simulink model "Foc_model_Matlab_obs"  (R2024b)
settings: Solver=FixedStepDiscrete  StartTime=0.0  StopTime=5  RelTol=1e-3  EnableMultiTasking=on
PreLoadFcn:
  | mcb_pmsm_foc_hall_S32K144EVB_data;
InitFcn:
  | mbd_s32k_consistency_checks(bdroot(gcs));
model workspace (MAT data in the model file):
  IDC_OVERCURRENT = Simulink.Parameter
  IDC_OVERCURRENT.Value = 2.3
  IDC_OVERCURRENT.Complexity = 'real'
  IDC_OVERCURRENT.Dimensions = [1 1]
  IDC_OVERCURRENT.DataType = 'single'
  VDC_OVERVOLTAGE = Simulink.Parameter
  VDC_OVERVOLTAGE.Value = 16
  VDC_OVERVOLTAGE.Complexity = 'real'
  VDC_OVERVOLTAGE.Dimensions = [1 1]
  VDC_OVERVOLTAGE.DataType = 'single'
  VDC_UNDERVOLTAGE = Simulink.Parameter
  VDC_UNDERVOLTAGE.Value = 8
  VDC_UNDERVOLTAGE.Complexity = 'real'
  VDC_UNDERVOLTAGE.Dimensions = [1 1]
  VDC_UNDERVOLTAGE.DataType = 'single'
undefined symbols (not defined in the file): DiscIntNeverNeededParam, External, inverter, Kcd, Kcq, Kid, Kiq, Kis, LQFP, mcb_isCodeGenVar, mcb_isSimVar, One, PI_params, pmsm, PU_System, Shot, sigbuilder_block, TRGMUX_PDB_TRIG, Ts, Ts_motor, Ts_simulink, Ts_speed
libraries: mbd_s32k1xx_ec_toolbox x35, mcbcontrolslib x8, simulink x6, mbd_msd_ec_toolbox x5, mcbpositiondecoderlib x3, hdlsllib x2, slpidlib x1, mcbsensorlessestimatorlib x1, mcbplantlib x1, autolibpmsmexterior x1, SignalEditorBlockLib x1
(part 1 of 2)
Description:
  | Field-Oriented Control for PMSM with Hall sensor with MTRDEVSPNK144.
  | This Simulink model is designed to work with Linix 45ZWN24-40 Motor and validate
  | that the motor can be rotated in closed loop with Hall sensor in Mathworks model from Motor Control Blockset.
  | The main scope of the model is to validate that the motor can run using Field-Oriented Control with Hall sensor.
  | 
  | FEATURES:
  | - Use FreeMASTER pannel to control the speed,
  | - Measure the 3-phase sinusoidal currents with PWM-PDB-ADC synchronization,
  | - Measure the DC bus voltage and current with PWM-PDB-ADC synchronization,
  | - PI Speed, Flux and Torque Controllers, position observer using Hall sensor.
  | 
  | HW SETUP:
  | - Configure S32K144 board supply voltage: J107:2-3(over USB),
  | - Configure J9,J10 and J11 on MotorGD: 2-3 (mode PMSM),
  | - Rotate trimmer resistor R72 (placed Devkit-MotorGD) counter-clockwise at maximum,
  | - Connect the motor phases to MotorGD J13 connector
  |   (i.e. Linix 45ZWN24-40: phA-white/phB-blue/phC-green),
  | - Power on the kit via J7 connector with 12Vdc.
  | 
  | VALIDATION:
  | - Run "mcb_pmsm_hall_offset_S32K144EVB_NXP.mdl" model to find out the position offset and
  | update it in "mcb_pmsm_foc_hall_S32K144EVB_data.m" script, run this script,
  | - Build/Simulate the model,
  | - After reset or power on, the Green LED shall be ON,
  | - In case of a FAULT the Red LED will be ON,
  | - Open FreeMASTER project and connect to the target.
  | - The initial speed command is set to 450rpm and can be changed from FreeMaster project.
  | - Click on the ON/OFF button to start then the speed of the motor it can be
  | changed using Speed gauge.
  | 
  | NOTE:
  | - In case of fault (RED LED is ON), the remove fault cause and press RESET button
  | 
  | Copyright (c) 2021 NXP
  | version 1.0.0
settings Model: Creator=nxf40284  LastModifiedBy=diego
settings SolverCC: AlgebraicLoopSolver=TrustRegion
settings DataIOCC: ExternalInput=off  InitialState=off  LimitDataPoints=on  SaveFormat=Array  SaveOutput=off  SaveTime=off  ReturnWorkspaceOutputs=off
settings OptimizationCC: DefaultParameterBehavior=Inlined  UseFloatMulNetSlope=on  DefaultUnderspecifiedDataType=single  UseSpecifiedMinMax=on  EnhancedBackFolding=on  PassReuseOutputArgsAs=Individual arguments  ZeroExternalMemoryAtStartup=off  ZeroInternalMemoryAtStartup=off  NoFixptDivByZeroProtection=on  EfficientFloat2IntCast=on  EfficientTunableParamExpr=on
settings DebuggingCC: AlgebraicLoopMsg=error  ArtificialAlgebraicLoopMsg=error  SolverPrmCheckMsg=warning  InheritedTsInSrcMsg=none  MultiTaskDSMMsg=none  MultiTaskCondExecSysMsg=none  TasksWithSamePriorityMsg=none  SigSpecEnsureSampleTimeMsg=none  ParameterPrecisionLossMsg=none  ParameterTunabilityLossMsg=error  FcnCallInpInsideContextMsg=warning  UnconnectedInputMsg=error  UnconnectedOutputMsg=error  UnconnectedLineMsg=error  AllowSymbolicDim=off  StateNameClashWarn=warning  SFUnexpectedBacktrackingDiag=warning  SFNoUnconditionalDefaultTransitionDiag=warning  SFExecutionAtInitializationDiag=none  ArithmeticOperatorsInVariantConditions=warning
settings HardwareCC: ProdBitPerPointer=32  ProdBitPerSizeT=32  ProdBitPerPtrDiffT=32  ProdLargestAtomicInteger=Long  ProdLargestAtomicFloat=Double  ProdWordSize=32  ProdHWDeviceType=ARM Compatible->ARM Cortex
settings ModelReferenceCC: EnableRefExpFcnMdlSchedulingChecks=on
settings SFSimCC: MATLABDynamicMemAlloc=off
settings RTWCC: Description=Model Based Design Toolbox S32K1xx Code Generation Target  SystemTargetFile=mbd_s32k.tlc  MakeCommand=mbd_s32k_make_rtw COPY_MDLREF_INCLUDES=0  TemplateMakefile=mbd_s32k.tmf  GenerateReport=on  IncludeHyperlinkInReport=on  GenerateTraceInfo=on  GenerateTraceReport=on  GenerateTraceReportSl=on  GenerateTraceReportSf=on  GenerateTraceReportEml=on  GPUComputeCapability=3.5
settings CodeAppCC: ForceParamTrailComments=on  IgnoreCustomStorageClasses=off  OperatorAnnotations=on  SimulinkDataObjDesc=on  SFDataObjDesc=on  InsertBlockDesc=on  StateflowObjectComments=on
settings STFCustomTargetCC: MultiwordLength=256  CombineOutputUpdateFcns=on  ERTCustomFileBanners=on  SupportContinuousTime=off  SupportNonInlinedSFcns=off  RemoveResetFunc=on  MATLABClassNameForMDSCustomization=Simulink.SoftwareTarget.ERTCustomization  SystemTargetFile=mbd_s32k.tlc
settings ERTTargetCC: ParMdlRefBuildCompliant=off  CompOptLevelCompliant=off  ConcurrentExecutionCompliant=off  ModelStepFunctionPrototypeControlCompliant=off  CPPClassGenCompliant=off  UseToolchainInfoCompliant=off  ERTSrcFileBannerTemplate=mbd_ert_code_template.cgt  ERTHdrFileBannerTemplate=mbd_ert_code_template.cgt  ERTDataSrcFileTemplate=mbd_ert_code_template.cgt  ERTDataHdrFileTemplate=mbd_ert_code_template.cgt  ERTCustomFileTemplate=example_file_process.tlc  ConvertIfToSwitch=off  SuppressUnreachableDefaultCases=off  DynamicArrayContainerType=coder::array

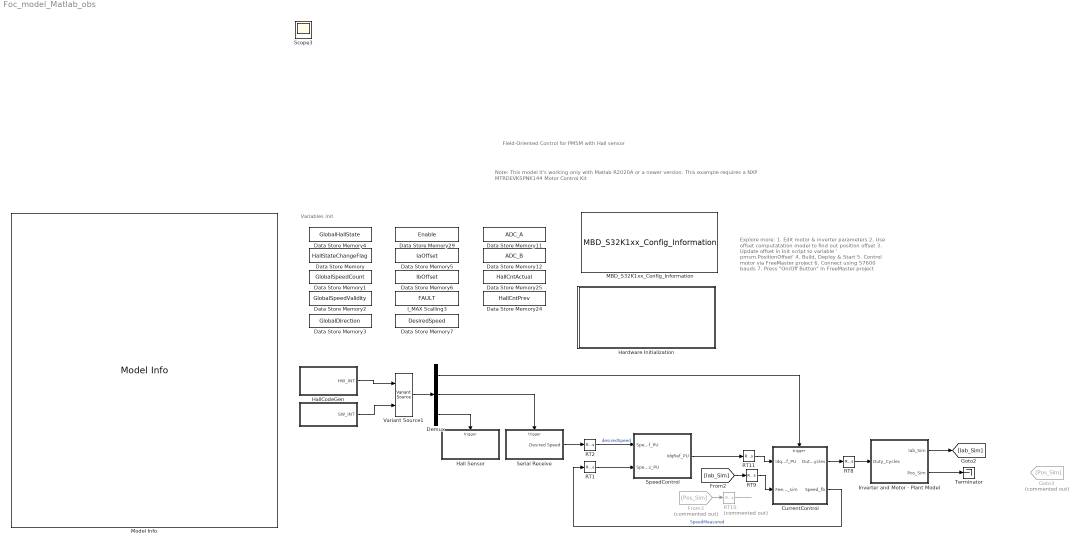
== system Foc_model_Matlab_obs ==
  note: Variables init
  note: Field-Oriented Control for PMSM with Hall sensor
  note: Explore more:
      | 1. Edit motor & inverter parameters
      | 2. Use offset computatation model to
      | find out position offset
      | 3. Update offset in Init script to variable ' pmsm.PositionOffset'
      | 4. Build, Deploy & Start
      | 5. Control motor via FreeMaster project
      | 6. Connect using 57600 bauds
      | 7. Press "On/Off Button" in FreeMaster project
  note: Note: This model it's working only with Matlab R2020A or a newer version.
      | This example requires a NXP MTRDEVKSPNK144 Motor Control Kit
  " " : Subsystem
  CurrentControl : Subsystem
      settings: RTWSystemCode=Nonreusable function  RTWFcnNameOpts=Use subsystem name
  Data Store Memory : DataStoreMemory  DataStoreName=HallStateChangeFlag  ShowAdditionalParam=off  OutDataTypeStr=uint16
  Data Store Memory1 : DataStoreMemory  DataStoreName=GlobalSpeedCount  ShowAdditionalParam=off  OutDataTypeStr=uint16
  Data Store Memory11 : DataStoreMemory  DataStoreName=ADC_A  ShowAdditionalParam=off
  Data Store Memory12 : DataStoreMemory  DataStoreName=ADC_B  ShowAdditionalParam=off
  Data Store Memory2 : DataStoreMemory  DataStoreName=GlobalSpeedValidity  ShowAdditionalParam=off  OutDataTypeStr=uint16
  Data Store Memory24 : DataStoreMemory  DataStoreName=HallCntPrev  ReadBeforeWriteMsg=warning  WriteAfterWriteMsg=warning  WriteAfterReadMsg=warning  ShowAdditionalParam=off  OutDataTypeStr=uint16
  Data Store Memory25 : DataStoreMemory  DataStoreName=HallCntActual  ReadBeforeWriteMsg=warning  WriteAfterWriteMsg=warning  WriteAfterReadMsg=warning  ShowAdditionalParam=off  OutDataTypeStr=uint16
  Data Store Memory29 : DataStoreMemory  DataStoreName=Enable  ShowAdditionalParam=off  OutDataTypeStr=boolean
  Data Store Memory3 : DataStoreMemory  DataStoreName=GlobalDirection  ShowAdditionalParam=off  OutDataTypeStr=int16
  Data Store Memory4 : DataStoreMemory  DataStoreName=GlobalHallState  ShowAdditionalParam=off  OutDataTypeStr=uint32
  Data Store Memory5 : DataStoreMemory  DataStoreName=IaOffset  InitialValue=inverter.CtSensAOffset  ShowAdditionalParam=off  OutDataTypeStr=single
  Data Store Memory6 : DataStoreMemory  DataStoreName=IbOffset  InitialValue=inverter.CtSensBOffset  ShowAdditionalParam=off  OutDataTypeStr=single
  Data Store Memory7 : DataStoreMemory  DataStoreName=DesiredSpeed  ReadBeforeWriteMsg=warning  WriteAfterWriteMsg=warning  WriteAfterReadMsg=warning  InitialValue=450  ShowAdditionalParam=off  OutDataTypeStr=single
  Demux : Demux  Outputs=3
  From3 : From  Commented=on  GotoTag=Pos_Sim
  Goto3 : Goto  Commented=on  GotoTag=Pos_Sim
  Hall Sensor : Subsystem
  HallCodeGen : Subsystem
  Hardware Initialization : Subsystem  Priority=2
  I_MAX Scalling3 : DataStoreMemory  Priority=0  DataStoreName=FAULT  ReadBeforeWriteMsg=warning  WriteAfterWriteMsg=warning  WriteAfterReadMsg=warning  ShowAdditionalParam=off  OutDataTypeStr=boolean
  Inverter and Motor - Plant Model : Subsystem
  MBD_S32K1xx_Config_Information : mbd_s32k1xx_ec_toolbox/MBD_S32K1xx_Config_Information  Priority=1  mbdt_ver=0  disp_str=|  config_params=[]  mcu_target_name=S32K144  mcu_target_package=100-LQFP  mcu_target_sram_size=64KB  mcu_system_clock_freq=80  mcu_xtal_freq=External 8  mcu_steptick_timer=LPIT Channel 0  mcu_steptick_prio=15  ds_import_enable=on  target_compiler=GCC  target_memory=FLASH  gcc_target_compile_opts=-mcpu=cortex-m4 -mthumb -mfloat-abi=hard -mfpu=fpv4-sp-d16 -O1 -g -gstrict-dwarf  gcc_target_assemble_opts=-mcpu=cortex-m4 -mthumb -mfloat-abi=hard -mfpu=fpv4-sp-d16 -g  gcc_target_link_opts=-mcpu=cortex-m4 -mthumb -mfloat-abi=hard -mfpu=fpv4-sp-d16  gcc_target_default_lcf=on  gcc_target_user_lcf=S32K144_64_flash.ld  ghs_target_compile_opts=-cpu=cortexm4f -thumb -DARM_MATH_CM4 -fpu=vfpv4_d16 -fsingle -Ogeneral -Wundef -Wimplicit-int -Wshadow -Wtrigraphs --no_commons --gnu_asm -gnu99 -gdwarf-2 -G  ghs_target_assemble_opts=-cpu=cortexm4f -fpu=vfpv4_d16  ghs_target_link_opts=-cpu=cortexm4f -thumb -fpu=vfpv4_d16  ghs_target_default_lcf=on  ghs_target_user_lcf=S32K144_64_flash.ld  iar_target_compile_opts=--cpu=Cortex-M4F --thumb --fpu=VFPv4_sp -Ol -e --debug --dlib_config normal  iar_target_assemble_opts=--cpu Cortex-M4F --thumb --fpu VFPv4_sp  iar_target_link_opts=--no_exceptions --vfe --inline  iar_target_default_lcf=on  iar_target_user_lcf=S32K144_64_flash.icf  pil_download_enable=off  rbl_download_enable=on  rbl_start_delay=5000  rbl_download_interface=OpenSDA  rbl_restart_request=off  rbl_com_port=Custom  rbl_com_port_custom=COM1  pil_download_rate=57600  pil_opensda_drive=Custom  pil_opensda_drive_custom=D  pil_uart_instance=1  pil_uart_rx=PTC6: [LPUART1_RX | Receive]  pil_uart_tx=PTC7: [LPUART1_TX | Transmit]  FTM_PWM_PcrCheckEnDis=on  FTM_Input_Edge_Inputs_PcrCheckEnDis=on  FTM_Dual_Edge_Inputs_PcrCheckEnDis=on  FTM_Quadrature_Inputs_PcrCheckEnDis=on  FTM_Hall_Sensor_Inputs_PcrCheckEnDis=on  LPTMR_PcrCheckEnDis=on  PIT_PcrCheckEnDis=on  RTC_PcrCheckEnDis=on  FlexCAN_PcrCheckEnDis=on  LIN_PcrCheckEnDis=on  FlexIO_PcrCheckEnDis=on  LPI2C_PcrCheckEnDis=on  LPSPI_PcrCheckEnDis=on  LPUART_PcrCheckEnDis=on  CMP_PcrCheckEnDis=on  GPIO_OutputPcrCheckEnDis=on  GPIO_InputPcrCheckEnDis=on  SBC_PcrCheckEnDis=on  BMS_PcrCheckEnDis=on  AMMCLIB_PcrCheckEnDis=on  FM_PcrCheckEnDis=on  Profile_PcrCheckEnDis=on  ConfigParams_PcrCheckEnDis=on  ModelRef_PcrCheckEnDis=on  PDB0_PcrCheckEnDis=on  CSEc_PcrCheckEnDis=on  eDMA_PcrCheckEnDis=on  FLASH_PcrCheckEnDis=on  ADC_PcrCheckEnDis=on  WDOG_PcrCheckEnDis=on
      | Target : S32K144-64KB_SRAM
      | Package : 100-pin
      | System clock : 80 MHz
      | XTAL clock : External 8 MHz
      | Compiler : IAR
      | Target Type : FLASH
      | Download Code after build : off
      | Step Tick Interrupt Priority : 15
  Model Info : simulink/Model-Wide Utilities/Model Info  Frame=off  DisplayStringWithTags=|  HorizontalTextAlignment=Left  LeftAlignmentValue=0.02
      | Model Name: %<ModelName>
      | 
      | Description: %<Description>
  RT1 : RateTransition  Priority=2  Deterministic=off  OutPortSampleTime=Ts_speed
  RT10 : RateTransition  Commented=on  Deterministic=off  OutPortSampleTime=Ts
  RT11 : RateTransition  Deterministic=off  OutPortSampleTime=Ts
  RT2 : RateTransition  Priority=1  Deterministic=off  OutPortSampleTime=Ts_speed
  RT8 : RateTransition  Deterministic=off
  RT9 : RateTransition  Deterministic=off  OutPortSampleTime=Ts
  Serial Receive : Subsystem  SystemSampleTime=1e-3
  SpeedControl : Subsystem  TreatAsAtomicUnit=on  SystemSampleTime=Ts_speed
      settings: RTWSystemCode=Nonreusable function  RTWFcnNameOpts=Use subsystem name
  Terminator : Terminator
  Variant Source1 : VariantSource
  Scope3 : Scope
  wires:
  " "/1(SW_INT) -> Variant Source1/2
  HallCodeGen/1(HW_INT) -> Variant Source1/1
  [Iab_Sim] -> RT9/1
  Serial Receive/1(Desired Speed) -> RT2/1
  RT9/1 -> CurrentControl/2(Feedbacks_sim)
  RT11/1 -> CurrentControl/1(Idq_ref_PU)
  From3/1 -> RT10/1
  RT10/1 -> ?
  SpeedControl/1(IdqRef_PU) -> RT11/1
  RT2/1 -> SpeedControl/1(Speed_Ref_PU)  "desiredSpeed"
  CurrentControl/1(Duty Cycles) -> RT8/1
  RT8/1 -> Inverter and Motor - Plant Model/1(Duty_Cycles)
  Inverter and Motor - Plant Model/2(Pos_Sim) -> Terminator/1
  Inverter and Motor - Plant Model/1(Iab_Sim) -> [Iab_Sim]
  RT1/1 -> SpeedControl/2(Speed_Meas_PU)
  CurrentControl/2(Speed_fb) -> RT1/1  "SpeedMeasured"
  Variant Source1/1 -> Demux/1
  Demux/3 -> Hall Sensor/Trigger
  Demux/2 -> Serial Receive/Trigger
  Demux/1 -> CurrentControl/Trigger

== system Foc_model_Matlab_obs/  ==
  CurrentController_INT : simulink/Ports & Subsystems/Function-Call Generator  sample_time=Ts  numberOfIterations=1  DisallowWideOutput=off
  Hall_INT : simulink/Ports & Subsystems/Function-Call Generator  sample_time=Ts  numberOfIterations=1  DisallowWideOutput=off
  Mux : Mux  Inputs=3
  SCI_Rx_INT : simulink/Ports & Subsystems/Function-Call Generator  sample_time=Ts  numberOfIterations=1  DisallowWideOutput=off
  SW_INT : Outport
  wires:
  Mux/1 -> SW_INT/1
  CurrentController_INT/1 -> Mux/1
  Hall_INT/1 -> Mux/3
  SCI_Rx_INT/1 -> Mux/2

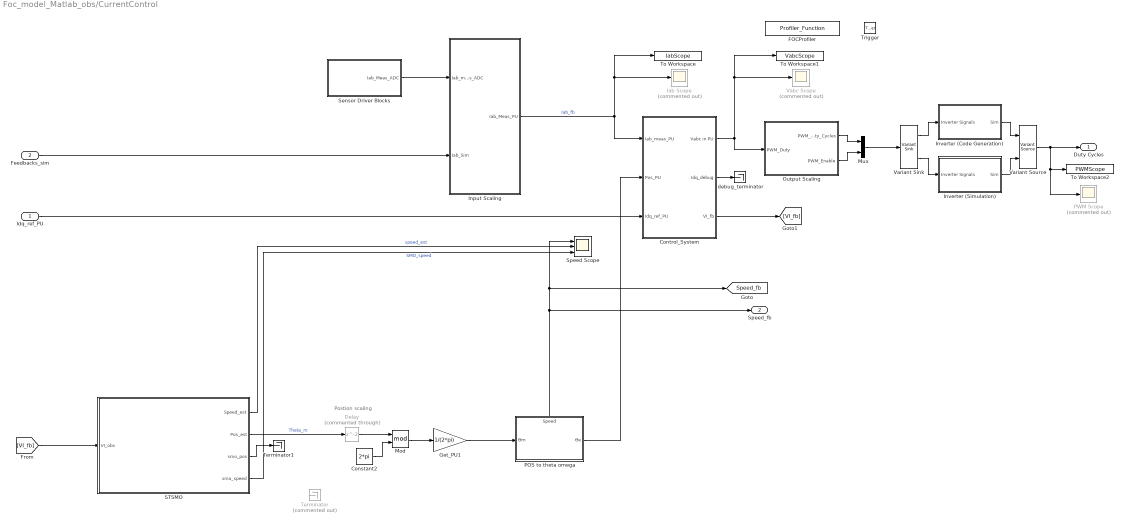
== system Foc_model_Matlab_obs/CurrentControl ==
  note: Postion scaling
  Idq_ref_PU : Inport
  Feedbacks_sim : Inport  Port=2
  Trigger : TriggerPort  TriggerType=function-call  VariantControl=Variant
  Constant2 : Constant  Value=2*pi  OutDataTypeStr=single  SampleTime=-1
  Control_System : Subsystem  Priority=3
  Delay : Delay  Commented=through
  FOCProfiler : mbd_s32k1xx_ec_toolbox/Utility Blocks/Profiler_Function  profile_indx=0
  Get_PU1 : Gain  Gain=1/(2*pi)  OutDataTypeStr=dataType  RndMeth=Simplest
  Iab Scope : Scope  Commented=on
  Input Scaling : Subsystem
  Inverter (Code Generation) : Subsystem  Priority=5
  Inverter (Simulation) : Subsystem
  Mod : Math  Operator=mod
  Mux : Mux  Inputs=2
  Output Scaling : Subsystem  Priority=4
  POS to theta omega : Subsystem
      settings: PortSchema="{\"entries\":[{\"content\":{\"sides\":[{\"content\":{\"connectorIds\":[\"In1\"]},\"type\":\"ConnectorPlacement.EquallySpacedRectSide\",\"uuid\":\"835816d9-4aa8-456c-963d-288b2d91bd0d\"},{\"content\":{\"connectorIds\":[\"Out1\"],\"side\":\"RIGHT\"},\"type\":\"ConnectorPlacement.EquallySpacedRectSide\",\"uuid\":\"100271e0-f614-4ef1-83bc-12c7604e80ba\"},{\"content\":{\"connectorIds\":[\"Out2\"],\"side\":\"TOP\"},\"type\":\"ConnectorPlacement.EquallySpacedRectSide\",\"uuid\":\"e3f4bec2-de67-41f7-95c5-b7e3793c521c\"}]},\"type\":\"ConnectorPlacement.EquallySpacedConnector\",\"uuid\":\"b67e7fce-f36c-4173-939b-340321a87f64\"}],\"packageUris\":[\"http://schema.mathworks.com/mf0/Connector/R2020b\"],\"version\":\"1.0\"}"
  PWM Scope : Scope  Commented=on
  STSMO : Subsystem
  Sensor Driver Blocks : Subsystem  Variant=on
  Speed Scope : Scope  NumInputPorts=3
  Terminator : Terminator  Commented=on
  Terminator1 : Terminator
  To Workspace : ToWorkspace  VariableName=IabScope  SaveFormat=Structure With Time  SampleTime=-1
  To Workspace1 : ToWorkspace  VariableName=VabcScope  SaveFormat=Structure With Time  SampleTime=-1
  To Workspace2 : ToWorkspace  VariableName=PWMScope  SaveFormat=Structure With Time  SampleTime=-1
  Vabc Scope : Scope  Commented=on
  Variant Sink : VariantSink
  Variant Source : VariantSource
  debug_terminator : Terminator
  Duty Cycles : Outport  InitialOutput=0  VectorParamsAs1DForOutWhenUnconnected=off
  Speed_fb : Outport  Port=2  InitialOutput=0  VectorParamsAs1DForOutWhenUnconnected=off
  tag scope: Speed_fb=global
  wires:
  Sensor Driver Blocks/1(Iab_Meas_ADC) -> Input Scaling/1(Iab_meas_ADC)
  Control_System/1(Vabc in PU) -> Output Scaling/1(PWM_Duty), To Workspace1/1, Vabc Scope/1
  Idq_ref_PU/1 -> Control_System/3(Idq_ref_PU)
  Input Scaling/1(Iab_Meas_PU) -> To Workspace/1, Iab Scope/1, Control_System/1(Iab_meas_PU)  "Iab_fb"
  Feedbacks_sim/1 -> Input Scaling/2(Iab_Sim)
  Output Scaling/1(PWM_Duty_Cycles) -> Mux/1
  Output Scaling/2(PWM_Enable) -> Mux/2
  Control_System/2(Idq_debug) -> debug_terminator/1
  Variant Sink/1 -> Inverter (Code Generation)/1(Inverter Signals)
  Inverter (Code Generation)/1(Sim) -> Variant Source/1
  Inverter (Simulation)/1(Sim) -> Variant Source/2
  Variant Sink/2 -> Inverter (Simulation)/1(Inverter Signals)
  Mux/1 -> Variant Sink/1
  Variant Source/1 -> To Workspace2/1, PWM Scope/1, Duty Cycles/1
  Control_System/3(VI_fb) -> [VI_fb]
  [VI_fb] -> STSMO/1(VI_obs)
  STSMO/3(smo_pos) -> Terminator1/1
  STSMO/4(smo_speed) -> Speed Scope/3  "SMO_speed"
  STSMO/1(Speed_est) -> Speed Scope/2  "speed_est"
  Constant2/1 -> Mod/2
  STSMO/2(Pos_est) -> Delay/1  "Theta_m"
  Mod/1 -> Get_PU1/1
  Get_PU1/1 -> POS to theta omega/1(ϴm)
  POS to theta omega/1(ϴe) -> Control_System/2(Pos_PU)
  POS to theta omega/2(Speed) -> Speed Scope/1, [Speed_fb], Speed_fb/1
  Delay/1 -> Mod/1

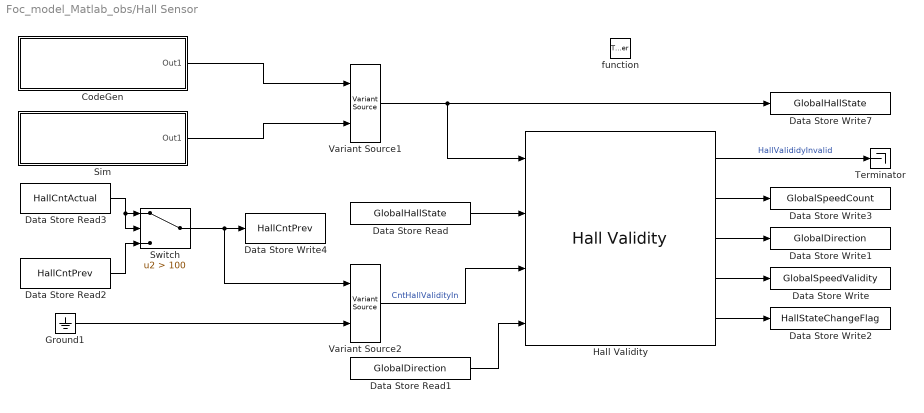
== system Foc_model_Matlab_obs/Hall Sensor ==
  function : TriggerPort  TriggerType=function-call  VariantControl=Variant
  CodeGen : Subsystem
  Data Store Read : DataStoreRead  Priority=1  DataStoreName=GlobalHallState  IndexOptions=Index vector (dialog)  Indices=1  OutputSizes=1
  Data Store Read1 : DataStoreRead  DataStoreName=GlobalDirection  IndexOptions=Index vector (dialog)  Indices=1  OutputSizes=1
  Data Store Read2 : DataStoreRead  DataStoreName=HallCntPrev  IndexOptions=Index vector (dialog)  Indices=1  OutputSizes=1
  Data Store Read3 : DataStoreRead  DataStoreName=HallCntActual  IndexOptions=Index vector (dialog)  Indices=1  OutputSizes=1
  Data Store Write : DataStoreWrite  DataStoreName=GlobalSpeedValidity  IndexOptions=Index vector (dialog)  Indices=1  OutputSizes=1
  Data Store Write1 : DataStoreWrite  DataStoreName=GlobalDirection  IndexOptions=Index vector (dialog)  Indices=1  OutputSizes=1
  Data Store Write2 : DataStoreWrite  DataStoreName=HallStateChangeFlag  IndexOptions=Index vector (dialog)  Indices=1  OutputSizes=1
  Data Store Write3 : DataStoreWrite  DataStoreName=GlobalSpeedCount  IndexOptions=Index vector (dialog)  Indices=1  OutputSizes=1
  Data Store Write4 : DataStoreWrite  DataStoreName=HallCntPrev  IndexOptions=Index vector (dialog)  Indices=1  OutputSizes=1
  Data Store Write7 : DataStoreWrite  Priority=2  DataStoreName=GlobalHallState  IndexOptions=Index vector (dialog)  Indices=1  OutputSizes=1
  Ground1 : Ground
  Hall Validity : mcbpositiondecoderlib/Hall Validity  hallSequence=CBA  sequence=[6,4,5,1,3,2]  CounterSize=16 bits
  Sim : Subsystem
  Switch : Switch  Criteria=u2 > Threshold  Threshold=100  SaturateOnIntegerOverflow=off  InputSameDT=off
  Terminator : Terminator
  Variant Source1 : VariantSource
  Variant Source2 : VariantSource
  wires:
  Hall Validity/3 -> Data Store Write1/1
  Hall Validity/5 -> Data Store Write2/1
  Hall Validity/4 -> Data Store Write/1
  Data Store Read1/1 -> Hall Validity/4
  Hall Validity/2 -> Data Store Write3/1
  Data Store Read/1 -> Hall Validity/2
  Hall Validity/1 -> Terminator/1  "HallValididyInvalid"
  Variant Source1/1 -> Hall Validity/1, Data Store Write7/1
  Ground1/1 -> Variant Source2/2
  Switch/1 -> Variant Source2/1, Data Store Write4/1
  Sim/1(Out1) -> Variant Source1/2
  CodeGen/1(Out1) -> Variant Source1/1
  Data Store Read2/1 -> Switch/3
  Data Store Read3/1 -> Switch/2, Switch/1
  Variant Source2/1 -> Hall Validity/3  "CntHallValidityIn"

== system Foc_model_Matlab_obs/HallCodeGen ==
  Data Store Write1 : DataStoreWrite  Priority=1  DataStoreName=HallCntActual  IndexOptions=Index vector (dialog)  Indices=1  OutputSizes=1
  FTM_Hall_Sensor : mbd_s32k1xx_ec_toolbox/Motor Control Blocks/FTM Blocks/FTM_Hall_Sensor  Priority=1  e_mode=Rising or Falling  prescaler=128  max_period=0.10486  isrlevel=5  mcuTargetUpdate=on  filter_en=off  filter_value=0  pinFtm1Ch1=PTA1: [FTM1_CH1 | FTM Channel]  pinFtm2Ch0=PTD10: [FTM2_CH0 | FTM Channel]  pinFtm2Ch1=PTD11: [FTM2_CH1 | FTM Channel]
  Mux : Mux  Inputs=3
  SCI_Rx_INT : simulink/Ports & Subsystems/Function-Call Generator  sample_time=0.1  numberOfIterations=1  DisallowWideOutput=off
  Subsystem2 : Subsystem  TreatAsAtomicUnit=on
  HW_INT : Outport
  wires:
  FTM_Hall_Sensor/2 -> Data Store Write1/1  "CntHall"
  Mux/1 -> HW_INT/1
  FTM_Hall_Sensor/1 -> Mux/3
  Subsystem2/1(FcnCall) -> Mux/1
  SCI_Rx_INT/1 -> Mux/2

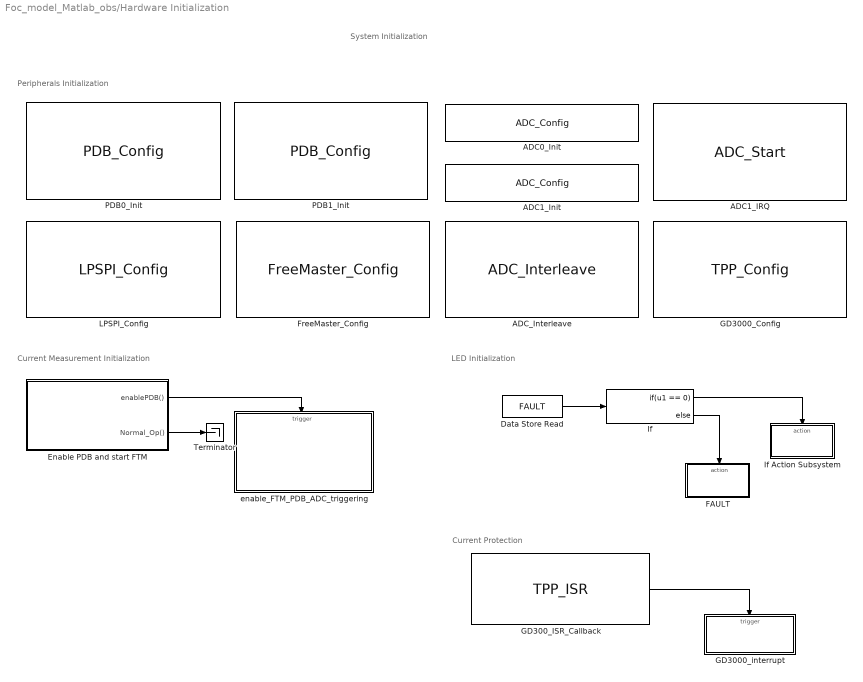
== system Foc_model_Matlab_obs/Hardware Initialization ==
  note: Peripherals Initialization
  note: System Initialization
  note: Current Measurement Initialization
  note: LED Initialization
  note: Current Protection
  ADC0_Init : mbd_s32k1xx_ec_toolbox/Motor Control Blocks/ADC Blocks/ADC_Config  Priority=3  instance=0  mode=12-bit conversion  smplts=2  adiclk=alternate clock 1  adiv=input clock  show_adv_opts=on  pretrgsel=PDB pre-trigger  swpretrg=Disabled  adtrg=hardware  trgsel=PDB output  refsel=Vrefh and Vrefl  supply_monitoring=off  acfe=off  acfgt=off  acren=off  cv1=0  cv2=0  adco=off  avge=off  avgs=4 samples
  ADC1_IRQ : mbd_s32k1xx_ec_toolbox/Motor Control Blocks/ADC Blocks/ADC_Start  Priority=5  instance=1  adc_r=C  adc_chan=PTB16: [ADC1_SE15 | ADC Single Ended Input]  aien=on  mcuTargetUpdate=on
  ADC1_Init : mbd_s32k1xx_ec_toolbox/Motor Control Blocks/ADC Blocks/ADC_Config  Priority=4  instance=1  mode=12-bit conversion  smplts=2  adiclk=alternate clock 1  adiv=input clock  show_adv_opts=on  pretrgsel=PDB pre-trigger  swpretrg=Disabled  adtrg=hardware  trgsel=PDB output  refsel=Vrefh and Vrefl  supply_monitoring=off  acfe=off  acfgt=off  acren=off  cv1=0  cv2=0  adco=off  avge=off  avgs=4 samples
  ADC_Interleave : mbd_s32k1xx_ec_toolbox/Motor Control Blocks/ADC Blocks/ADC_Interleave  adcInterleavePins=PTB1 to ADC0_SE5 and ADC1_SE15  adcInterleaveInit=on
  Data Store Read : DataStoreRead  DataStoreName=FAULT  IndexOptions=Index vector (dialog)  Indices=1  OutputSizes=1
  Enable PDB and start FTM : Stateflow chart  TreatAsAtomicUnit=on
  FAULT : Subsystem  TreatAsAtomicUnit=on
  FreeMaster_Config : mbd_s32k1xx_ec_toolbox/Utility Blocks/FreeMaster_Config  interface=LPUART1  baudrate=57600  rxd=PTC6: [LPUART1_RX | Receive]  txd=PTC7: [LPUART1_TX | Transmit]  mode=Short Interrupt  isr_prio=14  show_adv_opts=on  use_scope=on  max_scope_vars=8  use_recorder=on  max_rec_vars=8  rec_buff_size=8192  rec_timebase=100 microseconds  comm_buffer_size_auto=on  comm_buffer_size=255  comm_rqueue_size_default=on  comm_rqueue_size=32
  GD3000_Config : mbd_msd_ec_toolbox/TPP/TPP_Config  Priority=1  tppInstance=0  desatMode=on  fullonMode=off  lockMode=off  overtempEvent=on  phaseEvent=off  desatEvent=off  framingEvent=on  vlsEvent=on  writeErrEvent=on  overcurrentEvent=on  resetEvent=on  mcuTppIntEn=off  prioInt=15  tppDeadtime=500  initTppNow=on  tppSpiInst=0  tppPwmModule=3  tppPair0_1=on  tppPair2_3=on  tppPair4_5=on  tppPair6_7=off  tppFirstChHS=on  tppEn1Pin=PTA2: [PTA2 | Port A I/O]  tppEn2Pin=PTA2: [PTA2 | Port A I/O]  tppRstPin=PTA3: [PTA3 | Port A I/O]  tppCsPin=PTB5: [PTB5 | Port B I/O]  tppIntPin=PTE10: [PTE10 | Port E I/O]
  GD3000_interrupt : Subsystem  TreatAsAtomicUnit=on
  "GD300_ISR_Callback " : mbd_msd_ec_toolbox/TPP/TPP_ISR  tppInstance=0
  If : If  IfExpression=u1 == 0
  If Action Subsystem : Subsystem  TreatAsAtomicUnit=on
  "LPSPI_Config " : mbd_s32k1xx_ec_toolbox/Communication Blocks/SPI Blocks/LPSPI_Config   InstanceNumber=0  Role=Master  BaudRate=1000000  ShowAdvanced=on  sin=PTB3: [LPSPI0_SIN | LPSPI Serial Data Input]  sout=PTB4: [LPSPI0_SOUT | LPSPI Serial Data Output]  sck=PTB2: [LPSPI0_SCK | LPSPI Serial Clock I/O]  pcs0=None  pcs1=PTB5: [LPSPI0_PCS1 | Peripheral Chip Select 1]  pcs2=None  pcs3=None  CPHA=1  CPOL=0  BitOrder=MSB first  TransferSize=8  WhichPCS=0  PCSPol=ActiveLow  ContinuousTransfer=off
  PDB0_Init : mbd_s32k1xx_ec_toolbox/Motor Control Blocks/PDB Blocks/PDB_Config  Priority=1  pdbModule=0  regScCont=One-Shot  regScTrgsel=External (TRGMUX_PDB_TRIG)  trgMuxSel=FTM3 Initialize Trigger  trgMuxSelPin=PTB5: [TRGMUX_IN0 | Trigger Mux Input]  regModModulus=5000  regScPrescaler=1  regScMult=1  regPoenPoen0=off  regPo0DlyDly1=0  regPo0DlyDly2=0  enable_pdb_init=off  show_adv_opts=on  regCh0C1En0=on  regCh0C1En1=off  regCh0C1En2=off  regCh0C1En3=off  regCh0C1En4=off  regCh0C1En5=off  regCh0C1En6=off  regCh0C1En7=off  regCh0C1Bb0=off  regCh0C1Bb1=off  regCh0C1Bb2=off  regCh0C1Bb3=off  regCh0C1Bb4=off  regCh0C1Bb5=off  regCh0C1Bb6=off  regCh0C1Bb7=off  regCh0C1Tos0=Pre-trigger is in delay mode  regCh0C1Tos1=Pre-trigger is in delay mode  regCh0C1Tos2=Pre-trigger is in delay mode  regCh0C1Tos3=Pre-trigger is in delay mode  regCh0C1Tos4=Pre-trigger is in delay mode  regCh0C1Tos5=Pre-trigger is in delay mode  regCh0C1Tos6=Pre-trigger is in delay mode  regCh0C1Tos7=Pre-trigger is in delay mode  regCh0DlyDly0=2000  regCh0DlyDly1=0  regCh0DlyDly2=0  regCh0DlyDly3=0  regCh0DlyDly4=0  regCh0DlyDly5=0  regCh0DlyDly6=0  regCh0DlyDly7=0  regCh1C1En0=off  regCh1C1En1=off  regCh1C1En2=off  regCh1C1En3=off  regCh1C1En4=off  regCh1C1En5=off  regCh1C1En6=off  regCh1C1En7=off  regCh1C1Bb0=off  regCh1C1Bb1=off  regCh1C1Bb2=off  regCh1C1Bb3=off  regCh1C1Bb4=off  regCh1C1Bb5=off  regCh1C1Bb6=off  regCh1C1Bb7=off  regCh1C1Tos0=Pre-trigger is in delay mode  regCh1C1Tos1=Pre-trigger is in delay mode  regCh1C1Tos2=Pre-trigger is in delay mode  regCh1C1Tos3=Pre-trigger is in delay mode  regCh1C1Tos4=Pre-trigger is in delay mode  regCh1C1Tos5=Pre-trigger is in delay mode  regCh1C1Tos6=Pre-trigger is in delay mode  regCh1C1Tos7=Pre-trigger is in delay mode  regCh1DlyDly0=0  regCh1DlyDly1=0  regCh1DlyDly2=0  regCh1DlyDly3=0  regCh1DlyDly4=0  regCh1DlyDly5=0  regCh1DlyDly6=0  regCh1DlyDly7=0
  PDB1_Init : mbd_s32k1xx_ec_toolbox/Motor Control Blocks/PDB Blocks/PDB_Config  Priority=2  pdbModule=1  regScCont=One-Shot  regScTrgsel=External (TRGMUX_PDB_TRIG)  trgMuxSel=FTM3 Initialize Trigger  trgMuxSelPin=PTB5: [TRGMUX_IN0 | Trigger Mux Input]  regModModulus=5000  regScPrescaler=1  regScMult=1  regPoenPoen0=off  regPo0DlyDly1=0  regPo0DlyDly2=0  enable_pdb_init=off  show_adv_opts=on  regCh0C1En0=on  regCh0C1En1=on  regCh0C1En2=on  regCh0C1En3=off  regCh0C1En4=off  regCh0C1En5=off  regCh0C1En6=off  regCh0C1En7=off  regCh0C1Bb0=off  regCh0C1Bb1=off  regCh0C1Bb2=off  regCh0C1Bb3=off  regCh0C1Bb4=off  regCh0C1Bb5=off  regCh0C1Bb6=off  regCh0C1Bb7=off  regCh0C1Tos0=Pre-trigger is in delay mode  regCh0C1Tos1=Pre-trigger is in delay mode  regCh0C1Tos2=Pre-trigger is in delay mode  regCh0C1Tos3=Pre-trigger is in delay mode  regCh0C1Tos4=Pre-trigger is in delay mode  regCh0C1Tos5=Pre-trigger is in delay mode  regCh0C1Tos6=Pre-trigger is in delay mode  regCh0C1Tos7=Pre-trigger is in delay mode  regCh0DlyDly0=0  regCh0DlyDly1=1000  regCh0DlyDly2=2000  regCh0DlyDly3=0  regCh0DlyDly4=0  regCh0DlyDly5=0  regCh0DlyDly6=0  regCh0DlyDly7=0  regCh1C1En0=off  regCh1C1En1=off  regCh1C1En2=off  regCh1C1En3=off  regCh1C1En4=off  regCh1C1En5=off  regCh1C1En6=off  regCh1C1En7=off  regCh1C1Bb0=off  regCh1C1Bb1=off  regCh1C1Bb2=off  regCh1C1Bb3=off  regCh1C1Bb4=off  regCh1C1Bb5=off  regCh1C1Bb6=off  regCh1C1Bb7=off  regCh1C1Tos0=Pre-trigger is in delay mode  regCh1C1Tos1=Pre-trigger is in delay mode  regCh1C1Tos2=Pre-trigger is in delay mode  regCh1C1Tos3=Pre-trigger is in delay mode  regCh1C1Tos4=Pre-trigger is in delay mode  regCh1C1Tos5=Pre-trigger is in delay mode  regCh1C1Tos6=Pre-trigger is in delay mode  regCh1C1Tos7=Pre-trigger is in delay mode  regCh1DlyDly0=0  regCh1DlyDly1=0  regCh1DlyDly2=0  regCh1DlyDly3=0  regCh1DlyDly4=0  regCh1DlyDly5=0  regCh1DlyDly6=0  regCh1DlyDly7=0
  Terminator : Terminator
  enable_FTM_PDB_ADC_triggering : Subsystem  TreatAsAtomicUnit=on
      settings: RTWSystemCode=Inline
  wires:
  Enable PDB and start FTM/1(enablePDB()) -> enable_FTM_PDB_ADC_triggering/Trigger
  Enable PDB and start FTM/2(Normal_Op()) -> Terminator/1
  Data Store Read/1 -> If/1
  If/1 -> If Action Subsystem/Action
  "GD300_ISR_Callback "/1 -> GD3000_interrupt/Trigger
  If/2 -> FAULT/Action

== system Foc_model_Matlab_obs/Inverter and Motor - Plant Model ==
  Duty_Cycles : Inport
  Codegeneration : Subsystem
  Position Scope : Scope
  Simulation : Subsystem
  To Workspace : ToWorkspace  VariableName=PositionScope  SaveFormat=Structure With Time  SampleTime=-1
  Variant Sink : VariantSink
  Variant Source : VariantSource
  Variant Source1 : VariantSource
  Iab_Sim : Outport  VectorParamsAs1DForOutWhenUnconnected=off
  Pos_Sim : Outport  Port=2  VectorParamsAs1DForOutWhenUnconnected=off
  wires:
  Duty_Cycles/1 -> Variant Sink/1
  Variant Source/1 -> Iab_Sim/1
  Variant Source1/1 -> Pos_Sim/1
  Codegeneration/1(Iab_fb_Sim) -> Variant Source/1
  Codegeneration/2(Pos_fb_Sim) -> Variant Source1/1
  Variant Sink/1 -> Codegeneration/1(Duty_Cycles)
  Variant Sink/2 -> Simulation/1(Duty_Cycles)
  Simulation/1(Iab_fb_Sim) -> Variant Source/2
  Simulation/2(Pos_fb_Sim) -> Variant Source1/2, Position Scope/1, To Workspace/1

== system Foc_model_Matlab_obs/Serial Receive ==
  function : TriggerPort  TriggerType=function-call  VariantControl=Variant
  Code Generation : Subsystem
  Data Store Write : DataStoreWrite  DataStoreName=Enable  IndexOptions=Index vector (dialog)  Indices=1  OutputSizes=1
  Data Type Conversion3 : DataTypeConversion  OutDataTypeStr=boolean  RndMeth=Simplest  SaturateOnIntegerOverflow=off
  Demux : Demux  Outputs=2
  Simulation : Subsystem
  Variant Source : VariantSource
  Desired Speed : Outport  VectorParamsAs1DForOutWhenUnconnected=off
  wires:
  Code Generation/1(Data) -> Variant Source/1
  Simulation/1(Data) -> Variant Source/2
  Variant Source/1 -> Demux/1
  Data Type Conversion3/1 -> Data Store Write/1
  Demux/2 -> Data Type Conversion3/1
  Demux/1 -> Desired Speed/1

== system Foc_model_Matlab_obs/SpeedControl ==
  Speed_Ref_PU : Inport
  Speed_Meas_PU : Inport  Port=2
  FOCProfiler : mbd_s32k1xx_ec_toolbox/Utility Blocks/Profiler_Function  profile_indx=1
  Id_ref : Constant  Value=0  OutDataTypeStr=dataType  SampleTime=Ts_speed
  Mux : Mux  Inputs=2
  Mux1 : Mux  Inputs=2
  PI_Controller_Speed : Subsystem  Priority=2  TreatAsAtomicUnit=on
  Speed_Ref_Selector : Subsystem  Priority=1  TreatAsAtomicUnit=on
  To Workspace : ToWorkspace  VariableName=SpeedScope  SaveFormat=Structure With Time  SampleTime=-1
  speed scope : Scope  NumInputPorts=2
  IdqRef_PU : Outport  VectorParamsAs1DForOutWhenUnconnected=off
  wires:
  Speed_Meas_PU/1 -> Speed_Ref_Selector/2(Speed_Ref_Open), PI_Controller_Speed/2(N_fb), Mux/2, speed scope/2  "Speed_fb"
  Id_ref/1 -> Mux1/1
  Mux1/1 -> IdqRef_PU/1
  Speed_Ref_PU/1 -> Speed_Ref_Selector/1(Speed_Ref_In)  "Speed_Ref_PU"
  Speed_Ref_Selector/1(Speed_Ref_PU) -> PI_Controller_Speed/1(N_ref), speed scope/1, Mux/1  "Speed_Ref"
  PI_Controller_Speed/1(Iq_ref) -> Mux1/2  "Iq_ref"
  Mux/1 -> To Workspace/1

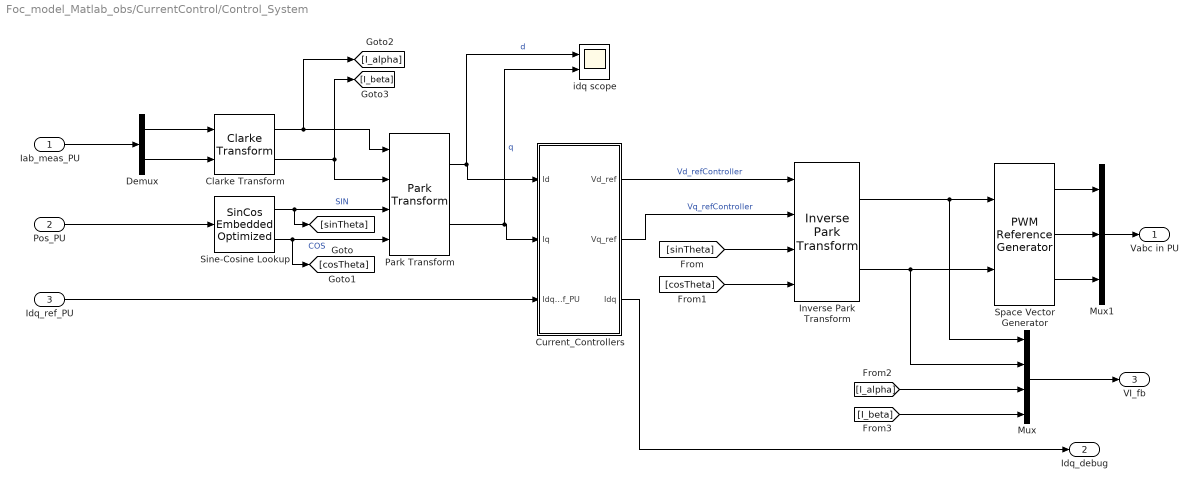
== system Foc_model_Matlab_obs/CurrentControl/Control_System ==
  Iab_meas_PU : Inport
  Pos_PU : Inport  Port=2
  Idq_ref_PU : Inport  Port=3
  Clarke Transform : mcbcontrolslib/Clarke Transform  VariantControl=Variant2  PhaseInput=Two inputs  EnPowerInv=off
  Current_Controllers : Subsystem
  Demux : Demux  Outputs=2
  Inverse Park Transform : mcbcontrolslib/Inverse Park Transform  PhaseInput=Two inputs  AxisAlignment=D-axis  ThetaInput=Sine and Cosine electrical position  AngleInput=Per-unit  N_points=1024
  Mux : Mux
  Mux1 : Mux  Inputs=3
  Park Transform : mcbcontrolslib/Park Transform  PhaseInput=Two inputs  AxisAlignment=D-axis  ThetaInput=Sine and Cosine electrical position  AngleInput=Per-unit  N_points=1024
  Sine-Cosine Lookup : mcbcontrolslib/SinCos Embedded Optimized  LabelModeActiveChoice=MCB_Sin  OptforProc=off  ApproximationMethod=None  UserApproxMethod=Lookup  ApproxStatus=None  InterpMethod=Linear point-slope  NumberOfDataPoints=16  NumberOfIterations=11  RemoveProtectionAgainstOutOfRangeInput=off  TableDataTypeStr=Inherit: Inherit via input  AngleInput=Per-unit  ThetaDataType=single  N_points=1024  DatatypeInput=Inherit from input  Datatype=Inherit: Same as input
  Space Vector Generator : mcbcontrolslib/PWM Reference Generator  inSignal=Valphabeta  modType=SVM: space vector modulation
  idq scope : Scope  NumInputPorts=2
  Vabc in PU : Outport  VectorParamsAs1DForOutWhenUnconnected=off
  Idq_debug : Outport  Port=2  VectorParamsAs1DForOutWhenUnconnected=off
  VI_fb : Outport  Port=3
  wires:
  Mux1/1 -> Vabc in PU/1
  [sinTheta] -> Inverse Park Transform/3
  Space Vector Generator/3 -> Mux1/3
  Space Vector Generator/1 -> Mux1/1
  Space Vector Generator/2 -> Mux1/2
  Idq_ref_PU/1 -> Current_Controllers/3(Idq_ref_PU)
  Iab_meas_PU/1 -> Demux/1
  Sine-Cosine Lookup/2 -> [cosTheta], Park Transform/4  "COS"
  Sine-Cosine Lookup/1 -> Park Transform/3, [sinTheta]  "SIN"
  Demux/1 -> Clarke Transform/1
  Demux/2 -> Clarke Transform/2
  Park Transform/2 -> idq scope/2, Current_Controllers/2(Iq)  "q"
  Park Transform/1 -> idq scope/1, Current_Controllers/1(Id)  "d"
  [cosTheta] -> Inverse Park Transform/4
  Current_Controllers/1(Vd_ref) -> Inverse Park Transform/1  "Vd_refController"
  Current_Controllers/2(Vq_ref) -> Inverse Park Transform/2  "Vq_refController"
  Pos_PU/1 -> Sine-Cosine Lookup/1
  Inverse Park Transform/1 -> Space Vector Generator/1, Mux/1
  Inverse Park Transform/2 -> Mux/2, Space Vector Generator/2
  Clarke Transform/1 -> [I_alpha], Park Transform/1
  Clarke Transform/2 -> [I_beta], Park Transform/2
  Current_Controllers/3(Idq) -> Idq_debug/1
  [I_beta] -> Mux/4
  [I_alpha] -> Mux/3
  Mux/1 -> VI_fb/1

== system Foc_model_Matlab_obs/CurrentControl/Input Scaling ==
  Iab_meas_ADC : Inport
  Iab_Sim : Inport  Port=2
  Read_Sensor (sim) : Subsystem  VariantControl=mcb_isSimVar()
  Iab_Meas_PU : Outport  VectorParamsAs1DForOutWhenUnconnected=off
  wires:
  Iab_meas_ADC/1 -> Read_Sensor (sim)/1(Iab_meas_ADC)
  Iab_Sim/1 -> Read_Sensor (sim)/2(Iab_Sim)
  Read_Sensor (sim)/1(Iab_Meas_PU) -> Iab_Meas_PU/1

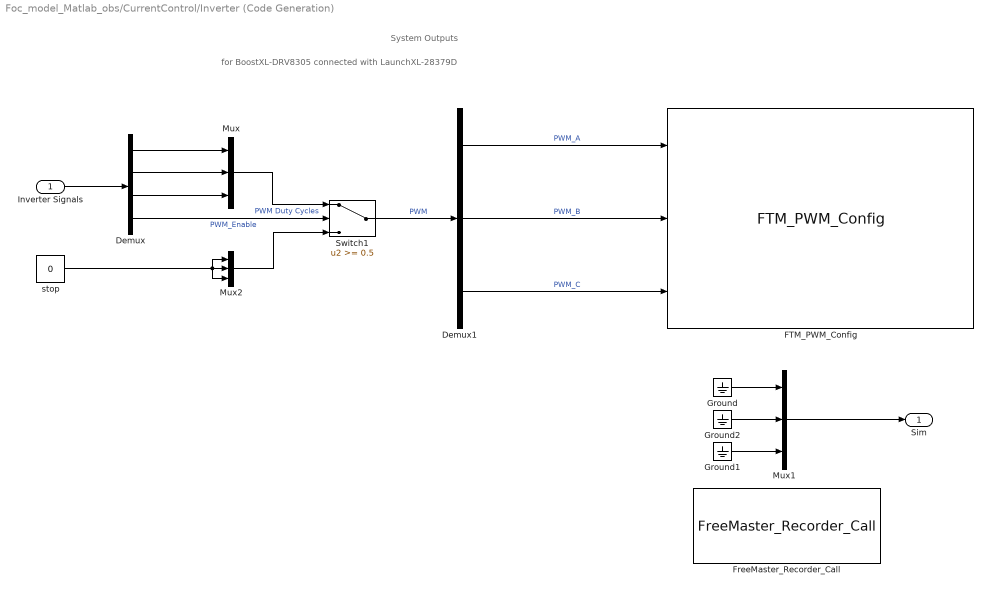
== system Foc_model_Matlab_obs/CurrentControl/Inverter (Code Generation) ==
  note: for BoostXL-DRV8305 connected with LaunchXL-28379D
  note: System Outputs
  Inverter Signals : Inport
  Demux : Demux
  Demux1 : Demux  Outputs=3
  FTM_PWM_Config : mbd_s32k1xx_ec_toolbox/Motor Control Blocks/FTM Blocks/FTM_PWM_Config  ftmModule=3  ftmMode=Center-Aligned PWM  ftmSourceClock=80 MHz  swcontrol_enable=off  chan0En=on  chan0Type=Complementary  chan2En=on  chan2Type=Complementary  chan4En=on  chan4Type=Complementary  chan6En=off  chan6Type=Independent  ftmPwmUnits=Hz  outFrequency=20000  ftmPeriod=4000  ftmPrescaler=Divide by 1  deadtimeUnits=Nanoseconds  deadtimeNs=0  deadtimeTicks=0  deadtimePrescaler=Divide by 1  dutyCycleCh0=0  dutyCycleCh1=0  dutyCycleCh2=0  dutyCycleCh3=0  dutyCycleCh4=0  dutyCycleCh5=0  dutyCycleCh6=0.25  dutyCycleCh7=0.25  dutyCycleSim=off  startAfterInit=off  showAdvOpt=on  pinFtmCh0=PTB8: [FTM3_CH0 | FTM Channel]  pinFtmCh1=PTB9: [FTM3_CH1 | FTM Channel]  pinPolCh0=Active Low  pinPolCh1=Active Low  outputComplem0=Main duplicated  outputLevel0=High  outputLevel1=Low  pinFtmCh2=PTB10: [FTM3_CH2 | FTM Channel]  pinFtmCh3=PTB11: [FTM3_CH3 | FTM Channel]  pinPolCh2=Active Low  pinPolCh3=Active Low  outputComplem2=Main duplicated  outputLevel2=High  outputLevel3=Low  pinFtmCh4=PTC10: [FTM3_CH4 | FTM Channel]  pinFtmCh5=PTC11: [FTM3_CH5 | FTM Channel]  pinPolCh4=Active Low  pinPolCh5=Active Low  outputComplem4=Main duplicated  outputLevel4=High  outputLevel5=Low  pinFtmCh6=PTC12: [FTM3_CH6 | FTM Channel]  pinFtmCh7=None  pinPolCh6=Active Low  pinPolCh7=Active Low  outputComplem6=Main duplicated  outputLevel6=Low  outputLevel7=Low  initTrigger=off  chTrigger0=off  chTrigger1=off  chTrigger2=off  chTrigger3=off  chTrigger4=off  chTrigger5=off  chTrigger6=off  chTrigger7=off  mcuTargetUpdate=on  pwmSyncTrg=Software trigger  pwmSyncHwRouting=TRGMUX_FTM7  pwmSyncTrg0=off  pwmSyncTrg1=off  pwmSyncTrg2=off  pwmSyncAutoClear=off  pwmSyncMinLoad=off  pwmSyncMaxLoad=on  pwmSyncInvert=PWM Syncronization  pwmSyncOutControl=PWM Syncronization  pwmSyncOutMask=PWM Syncronization  pwmSyncCounterInitial=PWM Syncronization  pwmSyncPoints=Wait Loading Points  reloadEnable=off  reloadPriority=15  reloadHalfCycle=off  reloadHCR=0  reloadFrequency=0  chnMatch0=off  chnMatch1=off  chnMatch2=off  chnMatch3=off  chnMatch4=off  chnMatch5=off  chnMatch6=off  chnMatch7=off  pwmFaultProtection=off  pwmFaultInterrupt=off  pwmFaultClearing=Fault control disabled  pwmFaultPinState=Safe Value  pwmFaultFilterValue=0  pwmFaultPriority=15  fault_disen_0=off  fault_filter_0=off  fault_polarity_0=Active High  fault_disen_1=off  fault_filter_1=off  fault_polarity_1=Active high  fault_disen_2=off  fault_filter_2=off  fault_polarity_2=Active high  fault_disen_3=off  fault_filter_3=off  fault_polarity_3=Active high  fault_pin_0=None  fault_pin_1=None  fault_pin_2=None  fault_pin_3=None
  FreeMaster_Recorder_Call : mbd_s32k1xx_ec_toolbox/Utility Blocks/FreeMaster_Recorder_Call
  Ground : Ground
  Ground1 : Ground
  Ground2 : Ground
  Mux : Mux  Inputs=3
  Mux1 : Mux  Inputs=3
  Mux2 : Mux  Inputs=3
  Switch1 : Switch  Threshold=0.5  SaturateOnIntegerOverflow=off  InputSameDT=off
  stop : Constant  Value=0  OutDataTypeStr=Inherit: Inherit via back propagation
  Sim : Outport  VectorParamsAs1DForOutWhenUnconnected=off
  wires:
  Mux/1 -> Switch1/1  "PWM Duty Cycles"
  Demux/1 -> Mux/1
  Demux/3 -> Mux/3
  stop/1 -> Mux2/3, Mux2/2, Mux2/1
  Mux2/1 -> Switch1/3
  Inverter Signals/1 -> Demux/1
  Demux/2 -> Mux/2
  Demux/4 -> Switch1/2  "PWM_Enable"
  Switch1/1 -> Demux1/1  "PWM"
  Demux1/1 -> FTM_PWM_Config/1  "PWM_A"
  Demux1/2 -> FTM_PWM_Config/2  "PWM_B"
  Demux1/3 -> FTM_PWM_Config/3  "PWM_C"
  Ground2/1 -> Mux1/2
  Ground1/1 -> Mux1/3
  Ground/1 -> Mux1/1
  Mux1/1 -> Sim/1

== system Foc_model_Matlab_obs/CurrentControl/Inverter (Simulation) ==
  Inverter Signals : Inport
  Data Type Duplicate : DataTypeDuplicate
  Demux : Demux
  Mux : Mux  Inputs=3
  Mux2 : Mux  Inputs=3
  Switch1 : Switch  Threshold=0.5  RndMeth=Simplest  SaturateOnIntegerOverflow=off  InputSameDT=off
  stop : Constant  Value=0  OutDataTypeStr=Inherit: Inherit via back propagation
  Sim : Outport  VectorParamsAs1DForOutWhenUnconnected=off
  wires:
  stop/1 -> Data Type Duplicate/2, Mux2/1, Mux2/3, Mux2/2
  Mux2/1 -> Switch1/3
  Switch1/1 -> Sim/1
  Inverter Signals/1 -> Demux/1
  Demux/4 -> Switch1/2  "PWM Enable"
  Mux/1 -> Data Type Duplicate/1, Switch1/1  "PWM Duty Cycles"
  Demux/1 -> Mux/1
  Demux/2 -> Mux/2
  Demux/3 -> Mux/3

== system Foc_model_Matlab_obs/CurrentControl/Output Scaling ==
  PWM_Duty : Inport
  Constant1 : Constant  OutDataTypeStr=Inherit: Inherit via back propagation
  Data Type Conversion : DataTypeConversion  OutDataTypeStr=dataType  SaturateOnIntegerOverflow=off  RndMeth=Floor
  Enable : DataStoreRead  DataStoreName=Enable  IndexOptions=Index vector (dialog)  Indices=1  OutputSizes=1
  Gain : Gain  Gain=0.5  OutDataTypeStr=Inherit: Inherit via back propagation  RndMeth=Simplest
  Sum1 : Sum  Inputs=|++  RndMeth=Simplest
  PWM_Duty_Cycles : Outport
  PWM_Enable : Outport  Port=2
  wires:
  Enable/1 -> Data Type Conversion/1  "PWM_En"
  Data Type Conversion/1 -> PWM_Enable/1
  Gain/1 -> PWM_Duty_Cycles/1  "PWM_Duty_Cycles"
  Sum1/1 -> Gain/1
  Constant1/1 -> Sum1/2
  PWM_Duty/1 -> Sum1/1

== system Foc_model_Matlab_obs/CurrentControl/POS to theta omega ==
  ϴm : Inport
  Mechanical to Electrical Position : mcbpositiondecoderlib/Mechanical to Electrical Position  PolePairsInputType=Specify via dialog  NrPP=pmsm.p  selectedRange=Per unit  MechOfstInputType=Specify via dialog  mechOffsetIn=0  maxAngleIn=1  InputDataType=dataType  VariantSelect=floating-point
  Speed Measurement : mcbpositiondecoderlib/Speed Measurement  PositionUnit=Per unit  PositionScalingDatatype=uint32  SpeedCalculationMode=Time interval for speed calculation  SampleTimeAsync=Ts  MaximumApplicationSpeed=6000  SpeedResolution=5e-6  DelayLength=10  MaximumMeasurableSpeed=29999  MeasurableSpeedResolution=1.397e-05  SpeedUnit=Per unit based on dialog  PerUnitSpeed=pmsm.N_max  SpeedDataType=single
  ϴe : Outport
  Speed : Outport  Port=2
  wires:
  Speed Measurement/1 -> Speed/1
  ϴm/1 -> Mechanical to Electrical Position/1, Speed Measurement/1
  Mechanical to Electrical Position/1 -> ϴe/1

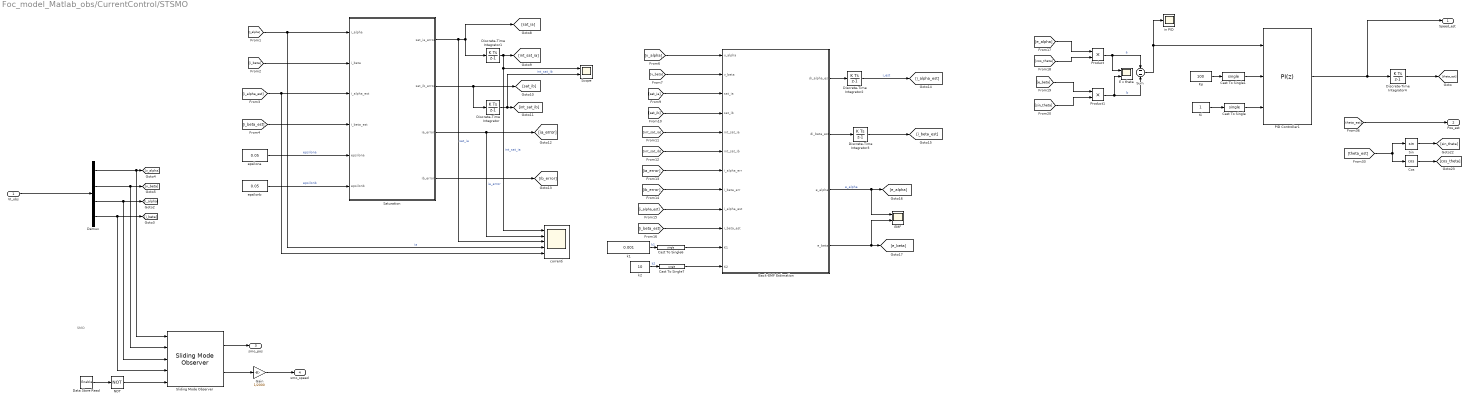
== system Foc_model_Matlab_obs/CurrentControl/STSMO ==
  note: SMO
  VI_obs : Inport
  Back-EMF Estimation : MATLAB Function  TreatAsAtomicUnit=on
  Cast To Single{,1,6..7} (4 alike) : DataTypeConversion  OutDataTypeStr=single  SaturateOnIntegerOverflow=off  RndMeth=Floor
  Cos : Trigonometry  Operator=cos
  Data Store Read : DataStoreRead  DataStoreName=Enable  IndexOptions=Index vector (dialog)  Indices=1  OutputSizes=1
  Demux : Demux
  Discrete-Time Integrator{,1..4} (5 alike) : DiscreteIntegrator  SampleTime=-1  ICPrevOutput=DiscIntNeverNeededParam  ICPrevScaledInput=DiscIntNeverNeededParam
  E x theta : Scope  NumInputPorts=2
  EMF : Scope  NumInputPorts=2
  Gain : Gain  Gain=1/2000
  Ki : Constant
  Kp : Constant  Value=100
  NOT : Logic  Operator=NOT  IconShape=distinctive  AllPortsSameDT=off  OutDataTypeStr=boolean
  PID Controller1 : slpidlib/PID Controller  Controller=PI  Form=Parallel  TimeDomain=Discrete-time  UseExternalTs=off  SampleTime=-1  IntegratorMethod=Forward Euler  FilterMethod=Forward Euler  ControllerParametersSource=external  P=1  I=1  UseKiTs=off  D=0  UseExternalDerivativeSource=off  N=100  UseFilter=on  TunerSelectOption=Transfer Function Based (PID Tuner App)  InitialConditionSource=internal  InitialConditionForIntegrator=0  InitialConditionForFilter=0  DifferentiatorICPrevScaledInput=0  ExternalReset=none  TrackingMode=off  Kt=1  LimitOutput=off  SatLimitsSource=internal  UpperSaturationLimit=inf  LowerSaturationLimit=-inf  LinearizeAsGain=on  AntiWindupMode=none  Kb=1  LimitIntegrator=off  UpperIntegratorSaturationLimit=inf  LowerIntegratorSaturationLimit=-inf  POutMin=[]  POutMax=[]  IOutMin=[]  IOutMax=[]  DOutMin=[]  DOutMax=[]  NOutMin=[]  NOutMax=[]  SumOutMin=[]  SumOutMax=[]  SaturationOutMin=[]  SaturationOutMax=[]  PParamMin=[]  PParamMax=[]  IParamMin=[]  IParamMax=[]  DParamMin=[]  DParamMax=[]  NParamMin=[]  NParamMax=[]  KbParamMin=[]  KbParamMax=[]  KtParamMin=[]  KtParamMax=[]  KbOutMin=[]  KbOutMax=[]  KtOutMin=[]  KtOutMax=[]  IntegratorOutMin=[]  IntegratorOutMax=[]  FilterOutMin=[]  FilterOutMax=[]  SumI1OutMin=[]  SumI1OutMax=[]  SumI2OutMin=[]  SumI2OutMax=[]  SumI3OutMin=[]  SumI3OutMax=[]  SumI4OutMin=[]  SumI4OutMax=[]  SumDOutMin=[]  SumDOutMax=[]  DifferentiatorOutMin=[]  DifferentiatorOutMax=[]  FilterDiffOutCoefMin=[]  FilterDiffOutCoefMax=[]  ReciprocalOutMin=[]  ReciprocalOutMax=[]  SumDenOutMin=[]  SumDenOutMax=[]  SumNumOutMin=[]  SumNumOutMax=[]  DivideOutMin=[]  DivideOutMax=[]  UdiffTsProdOutMin=[]  UdiffTsProdOutMax=[]  NTsProdOutMin=[]  NTsProdOutMax=[]  UintegralTsProdOutMin=[]  UintegralTsProdOutMax=[]  UngainTsProdOutMin=[]  UngainTsProdOutMax=[]  ClampingZeroOutDataTypeStr=Inherit: Inherit via back propagation  ClampingZeroOutMin=[]  ClampingZeroOutMax=[]  FilterDenConstantOutDataTypeStr=Inherit: Inherit via back propagation  FilterDenConstantOutMin=[]  FilterDenConstantOutMax=[]  PCopyOutDataTypeStr=Inherit: Inherit via back propagation  PCopyOutMin=[]  PCopyOutMax=[]  NCopyOutDataTypeStr=Inherit: Inherit via back propagation  NCopyOutMin=[]  NCopyOutMax=[]  IntegratorContinuousStateAttributes=''  IntegratorStateMustResolveToSignalObject=off  IntegratorRTWStateStorageClass=Auto  FilterContinuousStateAttributes=''  FilterStateMustResolveToSignalObject=off  FilterRTWStateStorageClass=Auto  ParallelPVariant=ExternalParameters  IdealPVariant=Disabled  IVariant=ExternalParameters  DVariant=Disabled  IntegratorVariant=Discrete  SatVariant=Disabled  AWVariant=Passthrough  PCopyVariant=Disabled  TRVariant=Disabled  FdbkBlocksVariant=Forward  IdealPFdbkVariant=Disabled  SatFdbkVariant=Disabled  DerivativeFilterVariant=Disabled  NVariant=Disabled  NCopyVariant=Disabled_SignalSpec  FilterICVariant=Disabled  IntegratorICVariant=InternalICs  ExternalResetVariant=Disabled  TRSumVariant=Passthrough  SumFdbkVariant=Disabled  SumVariant=Sum_PI  TsampFilterVariant=InternalTs  TsampNgainVariant=Passthrough  TsampIntegralVariant=Disabled_SignalSpec  ExternalSaturationOutDataTypeStr=Inherit: Same as second input  DerivativeSourceVariant=Disabled  PreIntVariant=InternalPreInt
  Product : Product
  Product1 : Product
  "Saturation " : MATLAB Function  TreatAsAtomicUnit=on
  Scope : Scope  NumInputPorts=2
  Sin : Trigonometry
  Sliding Mode Observer : mcbsensorlessestimatorlib/Sliding Mode Observer  InputUnit=Per-unit  BlkSampleTime=Ts  StatorResistance=pmsm.Rs  StatorInductance=pmsm.Ld  MaxApplicationSpeed=2500  PolePairs=pmsm.p  MaxStatorVoltage=PU_System.V_base  MaxStatorCurrent=PU_System.I_base  DisturbanceObserverGain=0.9  CurrentObserverGain=0.50881  CutoffFreq=1200  PositionUnit=Radians  PositionDataType=single  SpeedUnit=RPM  PerUnitSpeed=6000  SpeedDataType=single
  Sum : Sum  Inputs=--
  correnti : Scope  NumInputPorts=5
  epsilona : Constant  Value=0.05
  epsilonb : Constant  Value=0.05
  in PID : Scope
  k1 : Constant  Value=0.001
  k2 : Constant  Value=10
  Speed_est : Outport
  Pos_est : Outport  Port=2
  smo_pos : Outport  Port=3
  smo_speed : Outport  Port=4
  wires:
  Demux/4 -> Sliding Mode Observer/4, [i_beta]
  [i_beta] -> "Saturation "/2(i_beta)
  "Saturation "/1(sat_ia_error) -> correnti/3, Discrete-Time Integrator1/1, [sat_ia]  "sat_ia"
  "Saturation "/2(sat_ib_error) -> Discrete-Time Integrator/1, [sat_ib]
  "Saturation "/3(ia_error) -> correnti/2, [ia_error]  "ia_error"
  "Saturation "/4(ib_error) -> [ib_error]
  Discrete-Time Integrator/1 -> Scope/2, [int_sat_ib]  "int_sat_ib"
  Back-EMF Estimation/1(di_alpha_est) -> Discrete-Time Integrator2/1
  Back-EMF Estimation/2(di_beta_est) -> Discrete-Time Integrator3/1
  Back-EMF Estimation/3(e_alpha) -> EMF/1, [e_alpha]  "e_alpha"
  Back-EMF Estimation/4(e_beta) -> EMF/2, [e_beta]
  [v_alpha] -> Back-EMF Estimation/1(v_alpha)
  [v_beta] -> Back-EMF Estimation/2(v_beta)
  [sat_ia] -> Back-EMF Estimation/3(sat_ia)
  [sat_ib] -> Back-EMF Estimation/4(sat_ib)
  [int_sat_ia] -> Back-EMF Estimation/5(int_sat_ia)
  [int_sat_ib] -> Back-EMF Estimation/6(int_sat_ib)
  [ia_error] -> Back-EMF Estimation/7(i_alpha_err)
  [ib_error] -> Back-EMF Estimation/8(i_beta_err)
  [sin_theta] -> Product1/2
  [cos_theta] -> Product/2
  Discrete-Time Integrator4/1 -> [theta_est]
  VI_obs/1 -> Demux/1
  Sin/1 -> [sin_theta]
  Cos/1 -> [cos_theta]
  [theta_est] -> Pos_est/1
  k1/1 -> Cast To Single6/1  "k1"
  k2/1 -> Cast To Single7/1  "k2"
  epsilona/1 -> "Saturation "/5(epsilona)  "epsilona"
  epsilonb/1 -> "Saturation "/6(epsilonb)  "epsilonb"
  Demux/2 -> Sliding Mode Observer/2, [v_beta]
  Demux/1 -> Sliding Mode Observer/1, [v_alpha]
  Cast To Single6/1 -> Back-EMF Estimation/11(K1)
  Cast To Single7/1 -> Back-EMF Estimation/12(K2)
  Data Store Read/1 -> NOT/1
  NOT/1 -> Sliding Mode Observer/5
  Sliding Mode Observer/1 -> smo_pos/1
  Sliding Mode Observer/2 -> Gain/1
  Gain/1 -> smo_speed/1
  Demux/3 -> Sliding Mode Observer/3, [i_alpha]
  [i_alpha_est] -> Back-EMF Estimation/9(i_alpha_est)
  [i_beta_est] -> Back-EMF Estimation/10(i_beta_est)
  Product1/1 -> E x theta/2, Sum/2  "b"
  Discrete-Time Integrator3/1 -> [i_beta_est]
  Discrete-Time Integrator2/1 -> [i_alpha_est]  "i_est"
  PID Controller1/1 -> Speed_est/1, Discrete-Time Integrator4/1
  [e_beta] -> Product1/1
  [e_alpha] -> Product/1
  [i_beta_est] -> "Saturation "/4(i_beta_est)
  [i_alpha_est] -> correnti/5, "Saturation "/3(i_alpha_est)
  Ki/1 -> Cast To Single/1
  Kp/1 -> Cast To Single1/1
  [i_alpha] -> correnti/4, "Saturation "/1(i_alpha)  "ia"
  Discrete-Time Integrator1/1 -> correnti/1, Scope/1, [int_sat_ia]  "int_sat_ia"
  [theta_est] -> Sin/1, Cos/1
  Product/1 -> E x theta/1, Sum/1  "a"
  Cast To Single1/1 -> PID Controller1/2
  Sum/1 -> PID Controller1/1, in PID/1
  Cast To Single/1 -> PID Controller1/3

== system Foc_model_Matlab_obs/CurrentControl/Sensor Driver Blocks ==
  Sensor Driver Blocks (codegen) : Subsystem  VariantControl=mcb_isCodeGenVar()
  Sensor Driver Blocks (sim) : Subsystem  VariantControl=mcb_isSimVar()
  Iab_Meas_ADC : Outport
